simulink model "dof_dyn_pid_control_sim"  (R2019b)
settings: Solver=FixedStepAuto  StartTime=0.0  StopTime=63.05  FixedStep=h  RelTol=1e-3
values from neighbouring files (symbols this model uses):
  h = 0.1    [Example_9_Tracking_Delta_Input_Formulation.m]    (also in dyn_dist_mpc_control.m = 0.01; dyn_mpc_control.m = 0.01; dyn_pid_control.m = 0.01; init.m = 0.05)
  l_r = 100    [Copy_of_lateral_2_dof_model.m]    (also in init.m = 0.4125; init_scen_1.m = 0.4125; init_scen_3.m = 0.4125; lateral_2_dof_model.m = 0.4125)
  mass = evalin('base','mass')    [Nonlinear_model.m]    (also in init.m = 505; init_scen_1.m = 505; init_scen_3.m = 505; lateral_2_dof_model.m = 505)
  robot_vel = 3    [Example_9_Tracking_Delta_Input_Formulation.m]    (also in Nonlinear_model.m = evalin('base','robot_vel'); dyn_dist_mpc_control.m = 1; dyn_mpc_control.m = 1; dyn_pid_control.m = 1)
libraries: simulink x1, autolibshared x1
settings Model: Creator=faaizz  LastModifiedBy=faaizz
settings SFSimCC: CustomCodeUndefinedFunction=UseInterfaceOnly

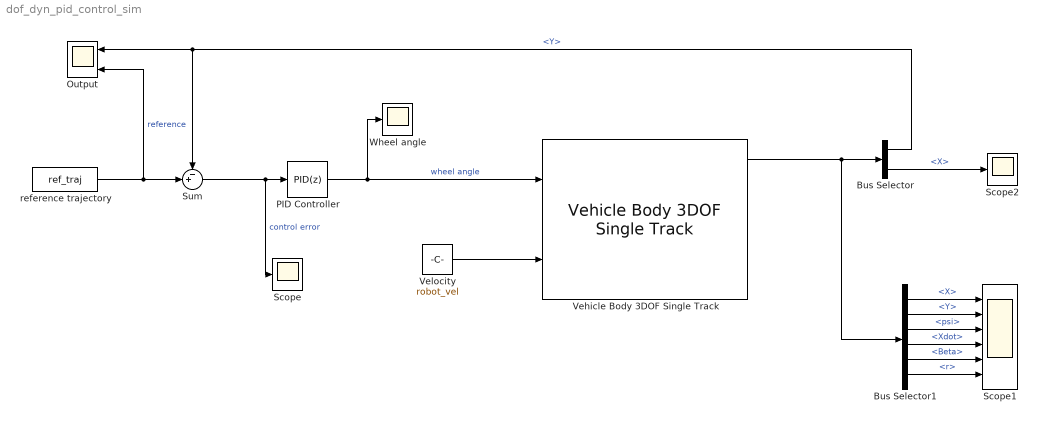
== system dof_dyn_pid_control_sim ==
  Bus Selector : BusSelector  OutputSignals=InertFrm.Cg.Disp.Y,InertFrm.Cg.Disp.X
  Bus Selector1 : BusSelector  OutputSignals=InertFrm.Cg.Disp.X,InertFrm.Cg.Disp.Y,InertFrm.Cg.Ang.psi,InertFrm.Cg.Vel.Xdot,BdyFrm.Cg.Ang.Beta,BdyFrm.Cg.AngVel.r
  Output : Scope  NumInputPorts=2
  PID Controller : simulink/Continuous/PID Controller  Controller=PID  Form=Parallel  TimeDomain=Discrete-time  SampleTime=h  IntegratorMethod=Forward Euler  FilterMethod=Forward Euler  ControllerParametersSource=internal  P=52.8226340320229  I=128.882425797399  D=0.37126334127225  UseFilter=on  N=187.558606068007  TunerSelectOption=Transfer Function Based (PID Tuner App)  InitialConditionSource=internal  InitialConditionForIntegrator=0  InitialConditionForFilter=0  DifferentiatorICPrevScaledInput=0  ExternalReset=none  TrackingMode=off  Kt=1  LimitOutput=off  UpperSaturationLimit=inf  LowerSaturationLimit=-inf  LinearizeAsGain=on  AntiWindupMode=none  Kb=1  POutMin=[]  POutMax=[]  IOutMin=[]  IOutMax=[]  DOutMin=[]  DOutMax=[]  NOutMin=[]  NOutMax=[]  SumOutMin=[]  SumOutMax=[]  SaturationOutMin=[]  SaturationOutMax=[]  PParamMin=[]  PParamMax=[]  IParamMin=[]  IParamMax=[]  DParamMin=[]  DParamMax=[]  NParamMin=[]  NParamMax=[]  KbParamMin=[]  KbParamMax=[]  KtParamMin=[]  KtParamMax=[]  KbOutMin=[]  KbOutMax=[]  KtOutMin=[]  KtOutMax=[]  IntegratorOutMin=[]  IntegratorOutMax=[]  FilterOutMin=[]  FilterOutMax=[]  SumI1OutMin=[]  SumI1OutMax=[]  SumI2OutMin=[]  SumI2OutMax=[]  SumI3OutMin=[]  SumI3OutMax=[]  SumI4OutMin=[]  SumI4OutMax=[]  SumDOutMin=[]  SumDOutMax=[]  DifferentiatorOutMin=[]  DifferentiatorOutMax=[]  FilterDiffOutCoefMin=[]  FilterDiffOutCoefMax=[]  ReciprocalOutMin=[]  ReciprocalOutMax=[]  SumDenOutMin=[]  SumDenOutMax=[]  SumNumOutMin=[]  SumNumOutMax=[]  DivideOutMin=[]  DivideOutMax=[]  IntegratorContinuousStateAttributes=''  IntegratorStateMustResolveToSignalObject=off  IntegratorRTWStateStorageClass=Auto  FilterContinuousStateAttributes=''  FilterStateMustResolveToSignalObject=off  FilterRTWStateStorageClass=Auto  ParallelPVariant=InternalParameters  IdealPVariant=Disabled  IVariant=InternalParameters  DVariant=InternalParameters  IntegratorVariant=Discrete  SatVariant=Disabled  AWVariant=Passthrough  PCopyVariant=Disabled  TRVariant=Disabled  FdbkBlocksVariant=Forward  IdealPFdbkVariant=Disabled  SatFdbkVariant=Disabled  DerivativeFilterVariant=ForwardEulerFilter  NVariant=InternalParameters  NCopyVariant=Disabled  FilterICVariant=InternalICsFilter  IntegratorICVariant=InternalICs  ExternalResetVariant=Disabled  TRSumVariant=Passthrough  SumFdbkVariant=Disabled  SumVariant=Sum_PID
  Scope : Scope
  Scope1 : Scope  NumInputPorts=6
  Scope2 : Scope
  Sum : Sum  Inputs=-+|
  Vehicle Body 3DOF Single Track : autolibshared/Vehicle Body 3DOF Single Track  trackMode=Single (bicycle)  inputMode=External longitudinal velocity  frontSteerMode=on  rearSteerMode=off  windMode=off  muMode=off  extFMode=off  extMMode=off  extXo=off  extpsio=off  extxdoto=off  extro=off  extYo=off  extTamb=off  extydoto=off  aMode=2  NF=1  NR=2  m=mass  a=l_f  b=l_r  h=0.3  X_o=0  xdot_o=0  CalphaMode=off  sigmaMode=on  d=0  w=[1.4,1.4]  Cy_f=C_f  Cy_r=C_r  sigma_f=.1  sigma_r=.1  alpha_f_brk=[-.1 .1]  Cy_f_data=[-9e3 9e3]  alpha_r_brk=[-.1 .1]  Cy_r_data=[-9e3 9e3]  Y_o=0  ydot_o=0  Izz=I_zz  psi_o=0  r_o=0  Af=2  Cd=.3  Cl=.1  Cpm=.1  beta_w=[0:0.01:0.3]  Cs=[0:0.03:0.9]  Cym=[0:0.01:0.3]  Pabs=101325  Tair=273  g=9.81  mu=1  xdot_tol=.01  Fznom=5000  Fxtire_sat=7e4  Fytire_sat=7e4  longOff=0  latOff=0  vertOff=0  wrapAng=off
      settings: SourceProductName=Powertrain Blockset  SourceProductBaseCode=PW
  Velocity : Constant  Value=robot_vel
  Wheel angle : Scope
  reference trajectory : FromWorkspace  VariableName=ref_traj  SampleTime=0  OutputAfterFinalValue=Setting to zero
  wires:
  reference trajectory/1 -> Sum/2, Output/2  "reference"
  Sum/1 -> Scope/1, PID Controller/1  "control error"
  PID Controller/1 -> Vehicle Body 3DOF Single Track/1, Wheel angle/1  "wheel angle"
  Vehicle Body 3DOF Single Track/1 -> Bus Selector1/1, Bus Selector/1
  Velocity/1 -> Vehicle Body 3DOF Single Track/2
  Bus Selector/1 -> Output/1, Sum/1  "<Y>"
  Bus Selector/2 -> Scope2/1  "<X>"
  Bus Selector1/1 -> Scope1/1  "<X>"
  Bus Selector1/2 -> Scope1/2  "<Y>"
  Bus Selector1/3 -> Scope1/3  "<psi>"
  Bus Selector1/4 -> Scope1/4  "<Xdot>"
  Bus Selector1/5 -> Scope1/5  "<Beta>"
  Bus Selector1/6 -> Scope1/6  "<r>"
